simulink model "plecs_PM5113_sim"  (R2015b)
settings: Solver=ode23s  StartTime=0.0  StopTime=0.1  RelTol=1e-3
undefined symbols (not defined in the file): plecs
libraries: plecslib x1, plecslib_extras x1
settings Model: ExtModeAutoUpdateStatusClock=off  Creator=hwolf  LastModifiedBy=kha
settings DataIOCC: LimitDataPoints=off  SaveFinalState=on  SaveFormat=Array  SignalLoggingSaveFormat=ModelDataLogs  SignalLoggingName=sigsOut
settings OptimizationCC: InitFltsAndDblsToZero=on
settings DebuggingCC: SaveWithParameterizedLinksMsg=none  UnderspecifiedInitializationDetection=Classic  MergeDetectMultiDrivingBlocksExec=none  SignalResolutionControl=TryResolveAllWithWarning  MultiTaskDSMMsg=warning  MultiTaskCondExecSysMsg=none
settings HardwareCC: ProdBitPerPointer=32  ProdLargestAtomicFloat=None  ProdIntDivRoundTo=Undefined  ProdEndianess=Unspecified  ProdWordSize=32  ProdHWDeviceType=32-bit Generic  TargetUnknown=on
settings GRTTargetCC: TargetFcnLib=ansi_tfl_tmw.mat  ModelReferenceCompliant=off  CombineOutputUpdateFcns=off  MatFileLogging=off  GRTInterface=on
settings ConfigComp: CovModelRefEnable=Off

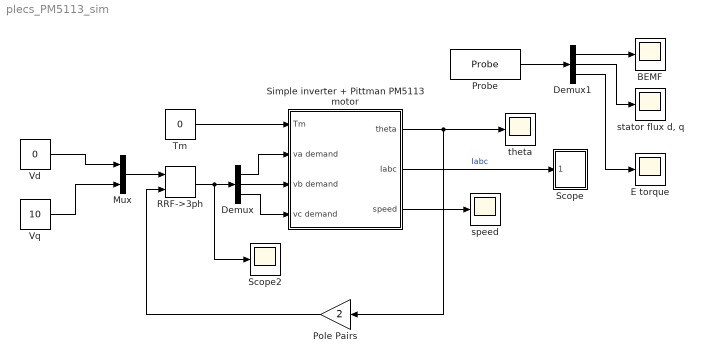
== system plecs_PM5113_sim ==
  BEMF : Scope
  Demux : Demux  Outputs=[1 1 1]
  Demux1 : Demux  Outputs=[3 2 1]
  E torque : Scope
  Mux : Mux  Inputs=2
  Pole Pairs : Gain  Gain=2
  Probe : plecslib/Probe  tagno=1
  RRF->3ph : plecslib_extras/Transformations/RRF->3ph
  Scope : Subsystem  LoadFcn=plecs('sl', 300);  InitFcn=plecs('sl', 314);  StartFcn=plecs('sl', 308);  StopFcn=plecs('sl', 309);  mask{Settings=<binary blob, 920 chars, not shown>}
      mask init:
      | plecsedit('sl', 315);
      settings: CopyFcn=plecs('sl', 303);  DeleteFcn=plecs('sl', 305);  UndoDeleteFcn=plecs('sl', 306);  PreSaveFcn=plecs('sl', 311);  NameChangeFcn=plecs('sl', 310);  DestroyFcn=plecs('sl', 307);  OpenFcn=plecs('sl', 302);  ErrorFcn=plerrorfcn
      mask Display: plot([0.1 0.9 0.9 0.1 0.1], [0.9 0.9 0.5 0.5 0.9])
  Scope2 : Scope
  Simple inverter + Pittman PM5113 motor : Subsystem  LoadFcn=plecs('sl', 200);  InitFcn=plecs('sl', 214);  StartFcn=plecs('sl', 208);  StopFcn=plecs('sl', 209);  mask(PlecsCircuit){PLECSData=<binary blob, 3356 chars, not shown>}
      mask prompts: PLECSData "PLECS Data (Do not delete or modify!)"
      mask help: Drag this block into a Simulink model to create a new electrical circuit.
      mask init:
      | % PLACE CUSTOM INITIALIZATIONS ABOVE
      | % DO NOT REMOVE
      | plecs('sl', 215);
      | % DO NOT REMOVE
      settings: CopyFcn=plecs('sl', 203);  DeleteFcn=plecs('sl', 205);  UndoDeleteFcn=plecs('sl', 206);  PreSaveFcn=plecs('sl', 211);  PostSaveFcn=plecs('sl', 201);  NameChangeFcn=plecs('sl', 210);  DestroyFcn=plecs('sl', 207);  PreCopyFcn=plecs('sl', 216);  OpenFcn=plecs('sl', 202);  ErrorFcn=plerrorfcn
      mask Display: disp('PLECS\nCircuit')
  Tm : Constant  Value=0
  Vd : Constant  Value=0
  Vq : Constant  Value=10
  speed : Scope
  "stator flux d, q" : Scope
  theta : Scope
  wires:
  Tm/1 -> Simple inverter + Pittman PM5113 motor/1(Tm)
  Simple inverter + Pittman PM5113 motor/1(theta) -> Pole Pairs/1, theta/1
  Pole Pairs/1 -> RRF->3ph/2
  RRF->3ph/1 -> Scope2/1, Demux/1
  Demux/1 -> Simple inverter + Pittman PM5113 motor/2(va demand)
  Demux/2 -> Simple inverter + Pittman PM5113 motor/3(vb demand)
  Demux/3 -> Simple inverter + Pittman PM5113 motor/4(vc demand)
  Mux/1 -> RRF->3ph/1
  Vd/1 -> Mux/1
  Vq/1 -> Mux/2
  Simple inverter + Pittman PM5113 motor/2(Iabc) -> Scope/1(1)  "Iabc"
  Probe/1 -> Demux1/1
  Demux1/1 -> BEMF/1
  Demux1/3 -> E torque/1
  Simple inverter + Pittman PM5113 motor/3(speed) -> speed/1
  Demux1/2 -> "stator flux d, q"/1

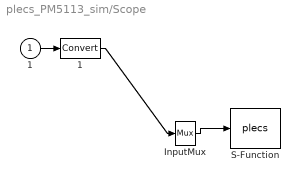
== system plecs_PM5113_sim/Scope ==
  1 : Inport
  " 1 " : DataTypeConversion  SaturateOnIntegerOverflow=on  RndMeth=Zero
  " InputMux " : Mux  Inputs=1
  " S-Function " : S-Function  FunctionName=plecs  SFunctionDeploymentMode=off  EnableBusSupport=off
  wires:
  " InputMux "/1 -> " S-Function "/1
  1/1 -> " 1 "/1
  " 1 "/1 -> " InputMux "/1

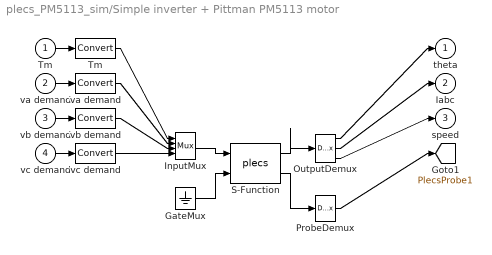
== system plecs_PM5113_sim/Simple inverter + Pittman PM5113 motor ==
  Tm : Inport  PortDimensions=1
  va demand : Inport  Port=2  PortDimensions=1
  vb demand : Inport  Port=3  PortDimensions=1
  vc demand : Inport  Port=4  PortDimensions=1
  " GateMux " : Ground
  " InputMux " : Mux  Inputs=[ 1 1 1 1 ]
  " OutputDemux " : Demux  Outputs=[ 1 3 1 ]
  " ProbeDemux " : Demux  Outputs=[ 6 ]
  " S-Function " : S-Function  FunctionName=plecs  SFunctionDeploymentMode=off  EnableBusSupport=off
  " Tm " : DataTypeConversion  SaturateOnIntegerOverflow=on  RndMeth=Zero
  " va demand " : DataTypeConversion  SaturateOnIntegerOverflow=on  RndMeth=Zero
  " vb demand " : DataTypeConversion  SaturateOnIntegerOverflow=on  RndMeth=Zero
  " vc demand " : DataTypeConversion  SaturateOnIntegerOverflow=on  RndMeth=Zero
  theta : Outport  PortDimensions=1
  Iabc : Outport  Port=2  PortDimensions=3
  speed : Outport  Port=3  PortDimensions=1
  tag scope: PlecsProbe1=global
  wires:
  " S-Function "/2 -> " ProbeDemux "/1
  " GateMux "/1 -> " S-Function "/2
  " InputMux "/1 -> " S-Function "/1
  " S-Function "/1 -> " OutputDemux "/1
  Tm/1 -> " Tm "/1
  " Tm "/1 -> " InputMux "/1
  va demand/1 -> " va demand "/1
  " va demand "/1 -> " InputMux "/2
  vb demand/1 -> " vb demand "/1
  " vb demand "/1 -> " InputMux "/3
  vc demand/1 -> " vc demand "/1
  " vc demand "/1 -> " InputMux "/4
  " OutputDemux "/1 -> theta/1
  " OutputDemux "/2 -> Iabc/1
  " OutputDemux "/3 -> speed/1
  " ProbeDemux "/1 -> [PlecsProbe1]
